simulink model "Music"  (R2020a)
settings: Solver=VariableStepAuto  StartTime=0.0  StopTime=Inf  RelTol=1e-3
libraries: dspmtrx3 x2, dspsnks4 x1, simulink x1, dspxfrm3 x1, dspvision x1, dspfdesign x1, dspstat3 x1
settings Model: Creator=albert  LastModifiedBy=albert

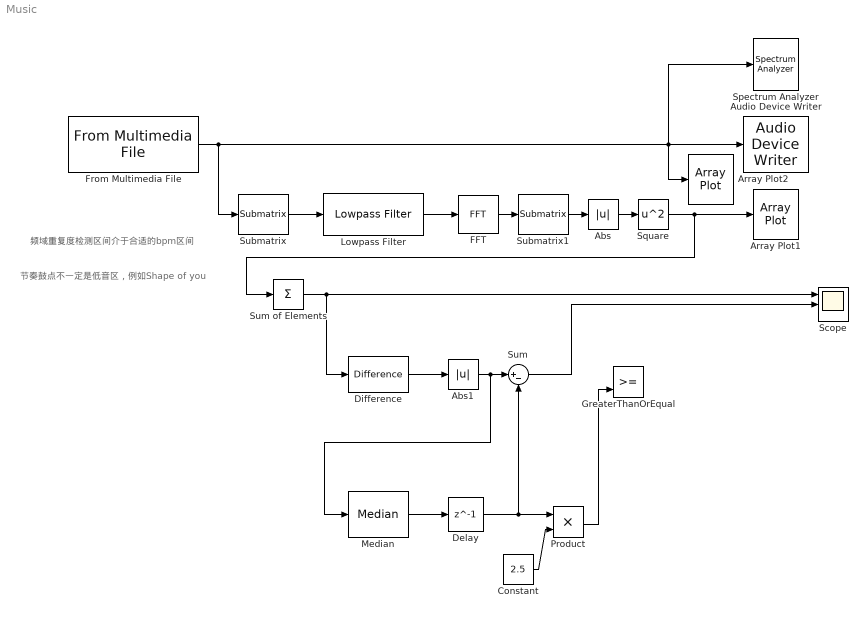
== system Music ==
  note: 节奏鼓点不一定是低音区，例如Shape of you
  note: 频域重复度检测区间介于合适的bpm区间
  Abs : Abs
  Abs1 : Abs
  Array Plot1 : ArrayPlot
  Array Plot2 : ArrayPlot
  Audio Device Writer : dspsnks4/Audio Device Writer  Driver=DirectSound  Device=Default  InheritSampleRate=on  SampleRate=44100  BitDepth=32-bit float  BufferSize=4096  NumBuffers=10  DefaultOutputChannelMapping=on  OutputChannelMapping=1:2  OutputNumUnderrunSamples=off  DriverIdx=1  DeviceWarnFlag=''
  Constant : Constant  Value=2.5
  Delay : Delay  DelayLength=1  InitialCondition=0
  Difference : simulink/Discrete/Difference  ICPrevInput=0.0  OutMin=[]  OutMax=[]  OutDataType=fixdt(1, 16)  OutScaling=2^-10  DoSatur=off
  FFT : dspxfrm3/FFT  FFTImplementation=Auto  CompMethod=Table lookup  TableOpt=NEW  TableOptActive=Speed  BitRevOrder=off  Normalize=on  InheritFFTLength=on  FFTLength=64  WrapInput=on  roundingMode=Floor  overflowMode=off  firstCoeffDataTypeStr=Inherit: Same word length as input  firstCoeffLastDataTypeStr=Inherit: Same word length as input  outputMin=[]  outputMax=[]
  From Multimedia File : dspvision/From Multimedia File  inputFilename=D:\CloudMusic\Ed Sheeran - Shape of You.flac  readRange=[1 Inf]  loop=on  numPlays=inf  outputStreams=Audio only  videoDataType=single  audioDataType=double  inheritSampleTime=on  userDefinedSampleTime=1/30  noAudioOutput=off  isIntensityVideo=off  fourcc=RGB  colorVideoFormat=Separate color signals  outputEOF=off  dataOrg=Column-major  audioFrameSize=1024  computeAudioFrameSize=off  outSamplingMode=Sample based
  GreaterThanOrEqual : RelationalOperator  OutDataTypeStr=fixdt(1,16)  RndMeth=Simplest
  Lowpass Filter : dspfdesign/Lowpass Filter  FilterType=IIR  DesignForMinimumOrder=on  FilterOrder=50  PassbandFrequency=100  StopbandFrequency=1000  PassbandRipple=0.1  StopbandAttenuation=80  InheritSampleRate=off  SampleRate=44100  SimulateUsing=Interpreted execution  roundingMode=Floor  coeffsDataTypeStr=fixdt(1,16)
  Median : dspstat3/Median  sortAlg=Quick sort  directionMode=Each column  dimension=1  roundingMode=Floor  overflowMode=off  accumDataTypeStr=Inherit: Same as product output  accumLastDataTypeStr=Inherit: Same as product output  outputDataTypeStr=Inherit: Same as accumulator  outputMin=[]  outputMax=[]  outputLastDataTypeStr=Inherit: Same as accumulator
      settings: SourceProductBaseCode=DS  allowOverrides=off
  Product : Product
  Scope : Scope  NumInputPorts=3
  Spectrum Analyzer : SpectrumAnalyzer
  Square : Math  Operator=square  SaturateOnIntegerOverflow=on
  Submatrix : dspmtrx3/Submatrix  RowSpan=Range of rows  RowStartMode=First  RowStartIndex=1  RowEndMode=Last  RowEndIndex=1  ColSpan=Range of columns  ColStartMode=Index  ColStartIndex=1  ColEndMode=Index  ColEndIndex=1
  Submatrix1 : dspmtrx3/Submatrix  RowSpan=Range of rows  RowStartMode=First  RowStartIndex=1  RowEndMode=Middle  RowEndIndex=1  ColSpan=Range of columns  ColStartMode=Index  ColStartIndex=1  ColEndMode=Index  ColEndIndex=1
  Sum : Sum  Inputs=|+-
  Sum of Elements : Sum  Inputs=+
  wires:
  From Multimedia File/1 -> Spectrum Analyzer/1, Array Plot2/1, Audio Device Writer/1, Submatrix/1
  FFT/1 -> Submatrix1/1
  Abs/1 -> Square/1
  Sum of Elements/1 -> Scope/1, Difference/1
  Difference/1 -> Abs1/1
  Abs1/1 -> Median/1, Sum/1
  Delay/1 -> Product/1, Sum/2
  Product/1 -> GreaterThanOrEqual/2
  Constant/1 -> Product/2
  Square/1 -> Array Plot1/1, Sum of Elements/1
  Submatrix/1 -> Lowpass Filter/1
  Submatrix1/1 -> Abs/1
  Lowpass Filter/1 -> FFT/1
  Sum/1 -> Scope/2
  Median/1 -> Delay/1
